simulink model "JointSpaceGravityCompensation"  (R2023a)
settings: Solver=VariableStepAuto  StartTime=0.0  StopTime=10.0  RelTol=1e-3
values from neighbouring files (symbols this model uses):
  Fc = 1    [parameters.m]
  Kd = [[60,0,0] ... (first row only)    [parameters.m]
  Kp = [[90,0,0] ... (first row only)    [parameters.m]
  qd = [pi/3, 0.1, 0.2]    [parameters.m]
settings Model: Creator=uzair  LastModifiedBy=syedj
settings OptimizationCC: ReuseModelBlockBuffer=off

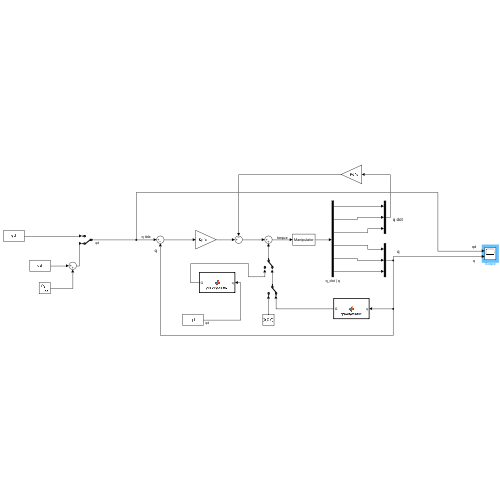
[thumbnail: Simulink's stored preview of the top-level diagram]
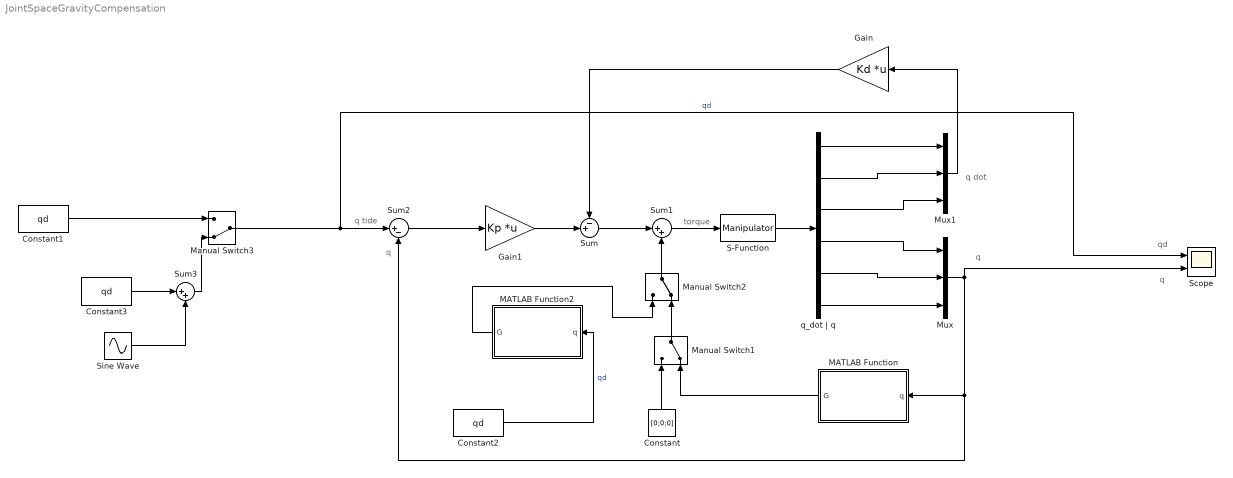
== system JointSpaceGravityCompensation ==
  note: q
  note: torque
  note: q tide
  note: q
  note: qd
  note: q
  note: q dot
  Constant : Constant  Value=[0;0;0]
  Constant1 : Constant  Value=qd
  Constant2 : Constant  Value=qd
  Constant3 : Constant  Value=qd
  Gain : Gain  Gain=Kd  Multiplication=Matrix(K*u)
  Gain1 : Gain  Gain=Kp  Multiplication=Matrix(K*u)
  MATLAB Function : MATLAB Function  TreatAsAtomicUnit=on
  MATLAB Function2 : MATLAB Function  TreatAsAtomicUnit=on
  Manual Switch1 : ManualSwitch  CurrentSetting=0
  Manual Switch2 : ManualSwitch  CurrentSetting=0
  Manual Switch3 : ManualSwitch  CurrentSetting=0
  Mux : Mux  Inputs=3
  Mux1 : Mux  Inputs=3
  S-Function : S-Function  FunctionName=Manipulator  Parameters=params  SFunctionDeploymentMode=off  EnableBusSupport=off
  Scope : Scope  NumInputPorts=2
  Sine Wave : Sin  Amplitude=0.1  Frequency=2*pi*Fc  SampleTime=0
  Sum : Sum  Inputs=-+|
  Sum1 : Sum  Inputs=|++
  Sum2 : Sum  Inputs=|+-
  Sum3 : Sum  Inputs=|++
  q_dot | q : Demux  Outputs=6
  wires:
  Manual Switch2/1 -> Sum1/2
  Manual Switch1/1 -> Manual Switch2/2
  Constant3/1 -> Sum3/1
  Manual Switch3/1 -> Scope/1, Sum2/1  "qd"
  Mux/1 -> Scope/2, Sum2/2, MATLAB Function/1(q)
  Constant1/1 -> Manual Switch3/1
  q_dot | q/3 -> Mux1/3
  Sine Wave/1 -> Sum3/2
  Sum2/1 -> Gain1/1
  Gain/1 -> Sum/1
  Mux1/1 -> Gain/1
  Constant/1 -> Manual Switch1/1
  q_dot | q/6 -> Mux/3
  q_dot | q/4 -> Mux/1
  MATLAB Function/1(G) -> Manual Switch1/2
  Sum1/1 -> S-Function/1
  Sum/1 -> Sum1/1
  Gain1/1 -> Sum/2
  q_dot | q/5 -> Mux/2
  Constant2/1 -> MATLAB Function2/1(q)  "qd"
  MATLAB Function2/1(G) -> Manual Switch2/1
  Sum3/1 -> Manual Switch3/2
  q_dot | q/2 -> Mux1/2
  S-Function/1 -> q_dot | q/1
  q_dot | q/1 -> Mux1/1

== matlab function JointSpaceGravityCompensation/MATLAB Function2 ==
  data: q input; G output; params parameter
function G = gravityMatrix(q, params)
    q1 = q(1);
    q2 = q(2);
    q3 = q(3);
    
    g = params.g;

    m1 = params.m(1);
    m2 = params.m(2);
    m3 = params.m(3);

    a1 = 0.02;
    a2 = 0.03;
    a3 = 0.01;
    b1 = 0.1256;
    b2 = 0.03;
    b3 = 0.01;
    c1 = 0.4;
    c2 = 0.46;
    c3 = 0.15;

    G = [(c1*g*m1*cos(q1))/2 + g*m2*cos(q1)*(c1 - c2/2) + g*m3*cos(q1)*(c1 + c3/2 + q3)
        0;
        g*m3*sin(q1)];
end

== matlab function JointSpaceGravityCompensation/MATLAB Function ==
  data: q input; G output; params parameter
function G = gravityMatrix(q, params)
    q1 = q(1);
    q2 = q(2);
    q3 = q(3);
    
    g = params.g;

    m1 = params.m(1);
    m2 = params.m(2);
    m3 = params.m(3);

    a1 = 0.02;
    a2 = 0.03;
    a3 = 0.01;
    b1 = 0.1256;
    b2 = 0.03;
    b3 = 0.01;
    c1 = 0.4;
    c2 = 0.46;
    c3 = 0.15;

    G = [(c1*g*m1*cos(q1))/2 + g*m2*cos(q1)*(c1 - c2/2) + g*m3*cos(q1)*(c1 + c3/2 + q3)
        0;
        g*m3*sin(q1)];
end
